simulink model "ProgettoControlli2_2"  (R2025b)
settings: Solver=VariableStepAuto  StartTime=0.0  StopTime=10.0  RelTol=1e-3
values from neighbouring files (symbols this model uses):
  a11 = -((h*S+(1/Rth))/Cth)    (= -2.41026145328)    [progetto.m]    (also in progetto_alternativo.m)
  a31 = (r1/r2)*((dlmax-(r1/r2)*z_star)/(m+(J/r2^2))) * dK_dx2    [progetto.m]    (also in progetto_alternativo.m)
  a32 = -((((r1)^2)*K)/(((r2)^2)*(m+(J/((r2)^2)))))    [progetto.m]    (also in progetto_alternativo.m)
  a33 = -(beta/(m+(J/((r2)^2))))    (= -0.576512455516)    [progetto.m]    (also in progetto_alternativo.m)
  b11 = 2*x1_eq/Cth    [progetto.m]    (also in progetto_alternativo.m)
  b12 = (h*S)/Cth    (= 0.0245945400968)    [progetto.m]    (also in progetto_alternativo.m)
  b13 = 1/(Cth*Rth)    (= 2.38566691319)    [progetto.m]    (also in progetto_alternativo.m)
  beta = 0.08    [progetto.m]    (also in progetto_alternativo.m)
  c = 6.2    [progetto.m]    (also in progetto_alternativo.m)
  Cth = 25.1 * 10^(-3)    (= 0.0251)    [progetto.m]    (also in progetto_alternativo.m)
  dlmax = l/100 * 4    (= 0.006)    [progetto.m]    (also in progetto_alternativo.m)
  g = 9.80665    [progetto.m]    (also in progetto_alternativo.m)
  h = 6.55    [progetto.m]    (also in progetto_alternativo.m)
  J = 2 * 10^(-4)    (= 0.0002)    [progetto.m]    (also in progetto_alternativo.m)
  K_max = 3.92 * 10^3    (= 3920)    [progetto.m]    (also in progetto_alternativo.m)
  m = 0.04    [progetto.m]    (also in progetto_alternativo.m)
  r1 = 0.0045    [progetto.m]    (also in progetto_alternativo.m)
  r2 = 0.045    [progetto.m]    (also in progetto_alternativo.m)
  Re = 4.8    [progetto.m]    (also in progetto_alternativo.m)
  Rth = 16.7    [progetto.m]    (also in progetto_alternativo.m)
  S = pi*d*l    (= 9.42477796077e-05)    [progetto.m]    (also in progetto_alternativo.m)
  Tamb = celsiusToKelvin(24)    [progetto.m]    (also in progetto_alternativo.m)
  Tavg = celsiusToKelvin(70)    [progetto.m]    (also in progetto_alternativo.m)
  Tdiff = 20    [progetto.m]    (also in progetto_alternativo.m)
  Tp = celsiusToKelvin(15)    [progetto.m]    (also in progetto_alternativo.m)
  x1_eq = sqrt((1/Re)*(h*S*(x2_eq - Tamb)+(x2_eq-Tp)/Rth))    [progetto.m]    (also in progetto_alternativo.m)
  x2_eq = Tavg + (Tdiff/c)*(log(K_star/(K_max - K_star)))    [progetto.m]    (also in progetto_alternativo.m)
  z_star = 0.04    [progetto.m]    (also in progetto_alternativo.m)
libraries: cstblocks x1
settings Model: Creator=nic  LastModifiedBy=nic

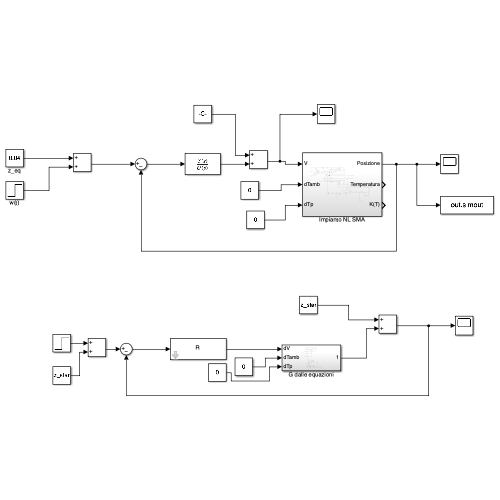
[thumbnail: Simulink's stored preview of the top-level diagram]
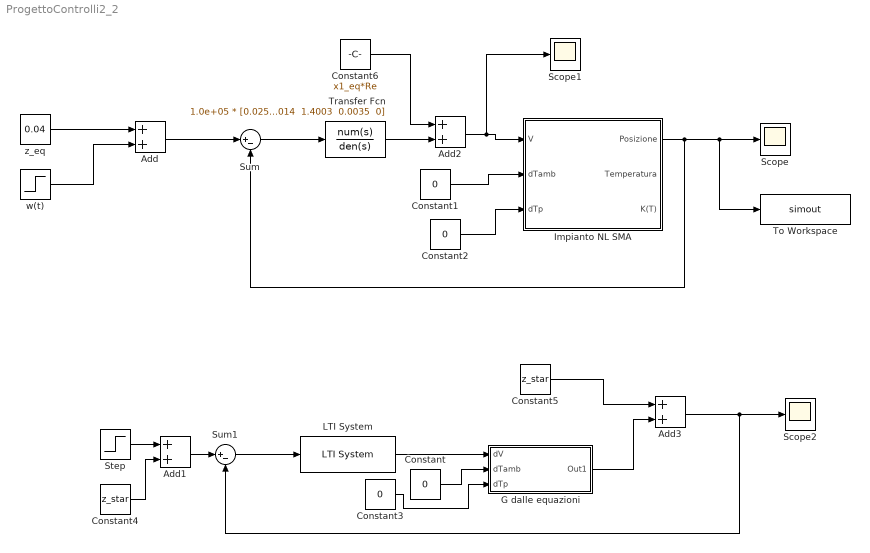
== system ProgettoControlli2_2 ==
  Add{,1..3} (4 alike) : Sum
  Constant{,1..3} (4 alike) : Constant  Value=0
  Constant4 : Constant  Value=z_star
  Constant5 : Constant  Value=z_star
  Constant6 : Constant  Value=x1_eq*Re
  G dalle equazioni : Subsystem
  Impianto NL SMA : Subsystem
  LTI System : cstblocks/LTI System  sys=R  IC=[]  PadeOrder=0
  Scope : Scope
      settings: ActiveDisplayYMinimum=0.030716392566077028  ActiveDisplayYMaximum=0.056016545973947569
  Scope1 : Scope
      settings: ActiveDisplayYMinimum=3.791369876272868  ActiveDisplayYMaximum=4.4632313606904432
  Scope2 : Scope
      settings: ActiveDisplayYMinimum=0.039693619486144291  ActiveDisplayYMaximum=0.046286194793895591  DataLoggingVariableName=ScopeData2
  Step : Step  Time=0  After=0.005  SampleTime=0
  Sum : Sum  Inputs=|+-
  Sum1 : Sum  Inputs=|+-
  To Workspace : ToWorkspace  VariableName=simout  SaveFormat=Timeseries  SampleTime=-1
  Transfer Fcn : TransferFcn  Numerator="1.0e+05 * [0.0250  0.0734  3.5752  7.8559  0.1749]"  Denominator="1.0e+04 * [0.0001  0.1014  1.4003  0.0035  0]"
  w(t) : Step  Time=5  After=0.005  SampleTime=0
  z_eq : Constant  Value=0.04
  wires:
  Constant1/1 -> Impianto NL SMA/2(dTamb)
  Constant2/1 -> Impianto NL SMA/3(dTp)
  z_eq/1 -> Add/1
  Impianto NL SMA/1(Posizione) -> Sum/2, To Workspace/1, Scope/1
  Add/1 -> Sum/1
  Sum/1 -> Transfer Fcn/1
  w(t)/1 -> Add/2
  Constant6/1 -> Add2/1
  Transfer Fcn/1 -> Add2/2
  Add2/1 -> Scope1/1, Impianto NL SMA/1(V)
  LTI System/1 -> G dalle equazioni/1(dV)
  Sum1/1 -> LTI System/1
  Constant/1 -> G dalle equazioni/2(dTamb)
  Constant3/1 -> G dalle equazioni/3(dTp)
  G dalle equazioni/1(Out1) -> Add3/2
  Step/1 -> Add1/1
  Add1/1 -> Sum1/1
  Constant4/1 -> Add1/2
  Constant5/1 -> Add3/1
  Add3/1 -> Scope2/1, Sum1/2

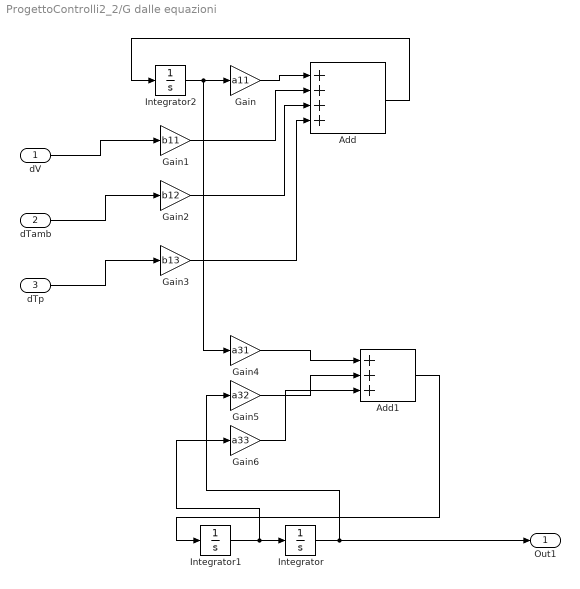
== system ProgettoControlli2_2/G dalle equazioni ==
  dV : Inport
  dTamb : Inport  Port=2
  dTp : Inport  Port=3
  Add : Sum  Inputs=++++
  Add1 : Sum  Inputs=+++
  Gain : Gain  Gain=a11
  Gain1 : Gain  Gain=b11
  Gain2 : Gain  Gain=b12
  Gain3 : Gain  Gain=b13
  Gain4 : Gain  Gain=a31
  Gain5 : Gain  Gain=a32
  Gain6 : Gain  Gain=a33
  Integrator : Integrator
  Integrator1 : Integrator
  Integrator2 : Integrator
  Out1 : Outport
  wires:
  Gain/1 -> Add/1
  dV/1 -> Gain1/1
  Gain1/1 -> Add/2
  dTamb/1 -> Gain2/1
  Gain2/1 -> Add/3
  dTp/1 -> Gain3/1
  Gain3/1 -> Add/4
  Add/1 -> Integrator2/1
  Integrator1/1 -> Gain6/1, Integrator/1
  Integrator2/1 -> Gain4/1, Gain/1
  Integrator/1 -> Out1/1, Gain5/1
  Gain4/1 -> Add1/1
  Gain5/1 -> Add1/2
  Add1/1 -> Integrator1/1
  Gain6/1 -> Add1/3

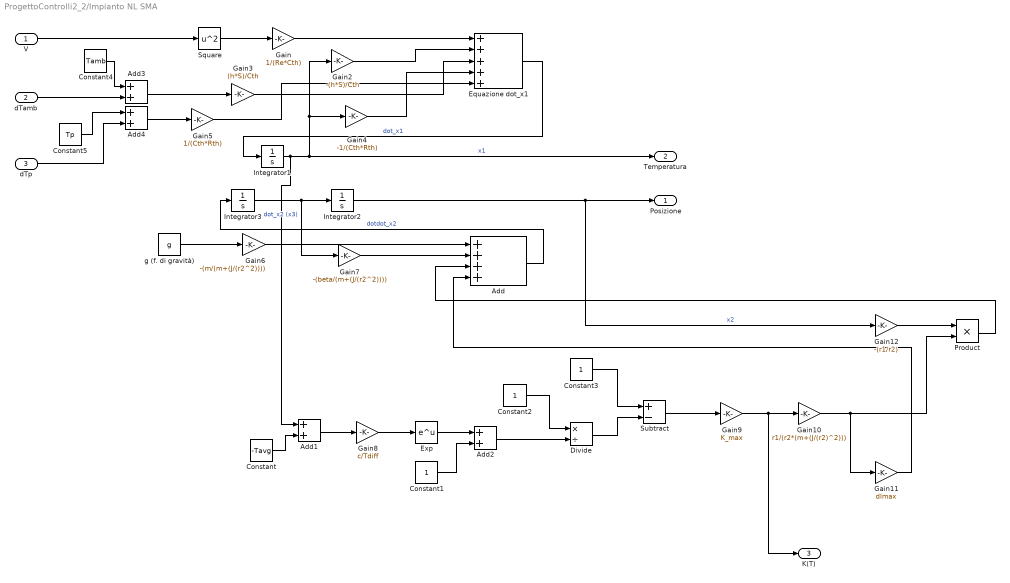
== system ProgettoControlli2_2/Impianto NL SMA ==
  V : Inport
  dTamb : Inport  Port=2
  dTp : Inport  Port=3
  Add : Sum  Inputs=++++
  Add{1..4} (4 alike) : Sum
  Constant : Constant  Value=-Tavg
  Constant1 : Constant
  Constant2 : Constant
  Constant3 : Constant
  Constant4 : Constant  Value=Tamb
  Constant5 : Constant  Value=Tp
  Divide : Product  Inputs=*/
  Equazione dot_x1 : Sum  Inputs=+++++
  Exp : Math
  Gain : Gain  Gain=1/(Re*Cth)
  Gain10 : Gain  Gain=r1/(r2*(m+(J/(r2)^2)))
  Gain11 : Gain  Gain=dlmax
  Gain12 : Gain  Gain=-(r1/r2)
  Gain2 : Gain  Gain=-(h*S)/Cth
  Gain3 : Gain  Gain=(h*S)/Cth
  Gain4 : Gain  Gain=-1/(Cth*Rth)
  Gain5 : Gain  Gain=1/(Cth*Rth)
  Gain6 : Gain  Gain=-(m/(m+(J/(r2^2))))
  Gain7 : Gain  Gain=-(beta/(m+(J/(r2^2))))
  Gain8 : Gain  Gain=c/Tdiff
  Gain9 : Gain  Gain=K_max
  Integrator1 : Integrator  InitialCondition=x2_eq
  Integrator2 : Integrator  InitialCondition=0.04
  Integrator3 : Integrator
  Product : Product
  Square : Math  Operator=square
  Subtract : Sum  Inputs=+-
  g (f. di gravità) : Constant  Value=g
  Posizione : Outport
  Temperatura : Outport  Port=2
  K(T) : Outport  Port=3
  wires:
  Add/1 -> Integrator3/1  "dotdot_x2"
  Square/1 -> Gain/1
  Integrator2/1 -> Gain12/1, Posizione/1  "x2"
  Exp/1 -> Add2/1
  Gain7/1 -> Add/2
  g (f. di gravità)/1 -> Gain6/1
  Gain11/1 -> Add/4
  Constant3/1 -> Subtract/1
  Gain/1 -> Equazione dot_x1/1
  Add1/1 -> Gain8/1
  Add2/1 -> Divide/2
  Gain9/1 -> K(T)/1, Gain10/1
  Integrator3/1 -> Gain7/1, Integrator2/1  "dot_x2 (x3)"
  Gain10/1 -> Gain11/1, Product/2
  Divide/1 -> Subtract/2
  Constant2/1 -> Divide/1
  Gain3/1 -> Equazione dot_x1/3
  Gain6/1 -> Add/1
  Constant/1 -> Add1/2
  Gain5/1 -> Equazione dot_x1/5
  Gain8/1 -> Exp/1
  Subtract/1 -> Gain9/1
  Gain2/1 -> Equazione dot_x1/2
  Integrator1/1 -> Add1/1, Temperatura/1, Gain4/1, Gain2/1  "x1"
  Gain12/1 -> Product/1
  Constant1/1 -> Add2/2
  Gain4/1 -> Equazione dot_x1/4
  Product/1 -> Add/3
  Equazione dot_x1/1 -> Integrator1/1  "dot_x1"
  dTamb/1 -> Add3/2
  Constant4/1 -> Add3/1
  Add3/1 -> Gain3/1
  Constant5/1 -> Add4/1
  Add4/1 -> Gain5/1
  dTp/1 -> Add4/2
  V/1 -> Square/1
